simulink model "ProcessModel_Boeing1"  (Simulink 7.9)
settings: Solver=VariableStepDiscrete  StartTime=0.0  StopTime=inf  RelTol=1e-3
libraries: simeventslib x43, simulink x1
settings Model: Creator=tsprock3  LastModifiedBy=tsprock3
settings DebuggingCC: UnconnectedInputMsg=none  UnconnectedOutputMsg=none  SimStateOlderReleaseMsg=warning

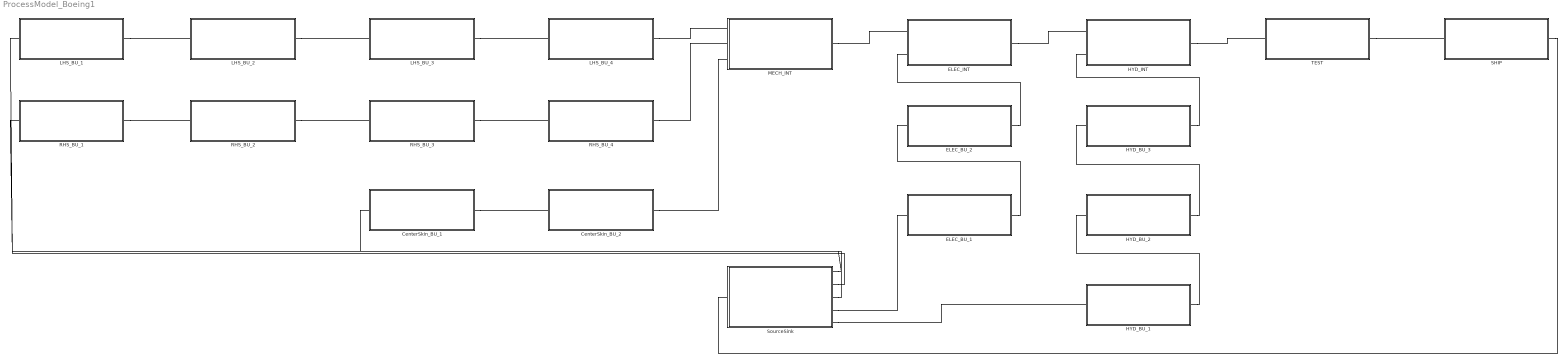
== system ProcessModel_Boeing1 ==
  CenterSkin_BU_1 : Subsystem
  CenterSkin_BU_2 : Subsystem
  ELEC_BU_1 : Subsystem
  ELEC_BU_2 : Subsystem
  ELEC_INT : Subsystem
  HYD_BU_1 : Subsystem
  HYD_BU_2 : Subsystem
  HYD_BU_3 : Subsystem
  HYD_INT : Subsystem
  LHS_BU_1 : Subsystem
  LHS_BU_2 : Subsystem
  LHS_BU_3 : Subsystem
  LHS_BU_4 : Subsystem
  MECH_INT : Subsystem
  RHS_BU_1 : Subsystem
  RHS_BU_2 : Subsystem
  RHS_BU_3 : Subsystem
  RHS_BU_4 : Subsystem
  SHIP : Subsystem
  SourceSink : Subsystem
  TEST : Subsystem
  connections:
  LHS_BU_1/RConn1 -- LHS_BU_2/LConn1
  LHS_BU_2/RConn1 -- LHS_BU_3/LConn1
  LHS_BU_3/RConn1 -- LHS_BU_4/LConn1
  RHS_BU_1/RConn1 -- RHS_BU_2/LConn1
  RHS_BU_2/RConn1 -- RHS_BU_3/LConn1
  RHS_BU_3/RConn1 -- RHS_BU_4/LConn1
  CenterSkin_BU_1/RConn1 -- CenterSkin_BU_2/LConn1
  LHS_BU_4/RConn1 -- MECH_INT/LConn1
  RHS_BU_4/RConn1 -- MECH_INT/LConn2
  CenterSkin_BU_2/RConn1 -- MECH_INT/LConn3
  MECH_INT/RConn1 -- ELEC_INT/LConn1
  ELEC_INT/RConn1 -- HYD_INT/LConn1
  ELEC_BU_1/RConn1 -- ELEC_BU_2/LConn1
  ELEC_BU_2/RConn1 -- ELEC_INT/LConn2
  HYD_BU_1/RConn1 -- HYD_BU_2/LConn1
  HYD_BU_2/RConn1 -- HYD_BU_3/LConn1
  HYD_BU_3/RConn1 -- HYD_INT/LConn2
  HYD_INT/RConn1 -- TEST/LConn1
  TEST/RConn1 -- SHIP/LConn1
  SourceSink/RConn1 -- LHS_BU_1/LConn1
  SourceSink/RConn2 -- RHS_BU_1/LConn1
  SourceSink/RConn3 -- CenterSkin_BU_1/LConn1
  SourceSink/RConn4 -- ELEC_BU_1/LConn1
  SourceSink/RConn5 -- HYD_BU_1/LConn1
  SHIP/RConn1 -- SourceSink/LConn1

== system ProcessModel_Boeing1/CenterSkin_BU_1 ==
  IN_Job : PathCombiner  NumberInputPorts=1
  OUT_Job : OutputSwitch  NumberOutputPorts=1
  Process : Subsystem
  IN_Job_1 : PMIOPort  Port=1  Side=Left
  OUT_Job_1 : PMIOPort  Port=2  Side=Right
  connections:
  Process/RConn1 -- OUT_Job/LConn1
  IN_Job/RConn1 -- Process/LConn1
  IN_Job/LConn1 -- IN_Job_1/RConn1
  OUT_Job/RConn1 -- OUT_Job_1/RConn1

== system ProcessModel_Boeing1/CenterSkin_BU_2 ==
  IN_Job : PathCombiner  NumberInputPorts=1
  OUT_Job : OutputSwitch  NumberOutputPorts=1
  Process : Subsystem
  IN_Job_1 : PMIOPort  Port=1  Side=Left
  OUT_Job_1 : PMIOPort  Port=2  Side=Right
  connections:
  Process/RConn1 -- OUT_Job/LConn1
  IN_Job/RConn1 -- Process/LConn1
  IN_Job/LConn1 -- IN_Job_1/RConn1
  OUT_Job/RConn1 -- OUT_Job_1/RConn1

== system ProcessModel_Boeing1/ELEC_BU_1 ==
  IN_Job : PathCombiner  NumberInputPorts=1
  OUT_Job : OutputSwitch  NumberOutputPorts=1
  Process : Subsystem
  IN_Job_1 : PMIOPort  Port=1  Side=Left
  OUT_Job_1 : PMIOPort  Port=2  Side=Right
  connections:
  Process/RConn1 -- OUT_Job/LConn1
  IN_Job/RConn1 -- Process/LConn1
  IN_Job/LConn1 -- IN_Job_1/RConn1
  OUT_Job/RConn1 -- OUT_Job_1/RConn1

== system ProcessModel_Boeing1/ELEC_BU_2 ==
  IN_Job : PathCombiner  NumberInputPorts=1
  OUT_Job : OutputSwitch  NumberOutputPorts=1
  Process : Subsystem
  IN_Job_1 : PMIOPort  Port=1  Side=Left
  OUT_Job_1 : PMIOPort  Port=2  Side=Right
  connections:
  Process/RConn1 -- OUT_Job/LConn1
  IN_Job/RConn1 -- Process/LConn1
  IN_Job/LConn1 -- IN_Job_1/RConn1
  OUT_Job/RConn1 -- OUT_Job_1/RConn1

== system ProcessModel_Boeing1/ELEC_INT ==
  IN_Job : EntityCombiner  NumberInputPorts=2  RetainComponentEntities=off
  OUT_Job : OutputSwitch  NumberOutputPorts=1
  Process : Subsystem
  IN_Job_1 : PMIOPort  Port=1  Side=Left
  IN_Job_2 : PMIOPort  Port=2  Side=Left
  OUT_Job_1 : PMIOPort  Port=3  Side=Right
  connections:
  Process/RConn1 -- OUT_Job/LConn1
  IN_Job/RConn1 -- Process/LConn1
  IN_Job/LConn1 -- IN_Job_1/RConn1
  IN_Job/LConn2 -- IN_Job_2/RConn1
  OUT_Job/RConn1 -- OUT_Job_1/RConn1

== system ProcessModel_Boeing1/HYD_BU_1 ==
  IN_Job : PathCombiner  NumberInputPorts=1
  OUT_Job : OutputSwitch  NumberOutputPorts=1
  Process : Subsystem
  IN_Job_1 : PMIOPort  Port=1  Side=Left
  OUT_Job_1 : PMIOPort  Port=2  Side=Right
  connections:
  Process/RConn1 -- OUT_Job/LConn1
  IN_Job/RConn1 -- Process/LConn1
  IN_Job/LConn1 -- IN_Job_1/RConn1
  OUT_Job/RConn1 -- OUT_Job_1/RConn1

== system ProcessModel_Boeing1/HYD_BU_2 ==
  IN_Job : PathCombiner  NumberInputPorts=1
  OUT_Job : OutputSwitch  NumberOutputPorts=1
  Process : Subsystem
  IN_Job_1 : PMIOPort  Port=1  Side=Left
  OUT_Job_1 : PMIOPort  Port=2  Side=Right
  connections:
  Process/RConn1 -- OUT_Job/LConn1
  IN_Job/RConn1 -- Process/LConn1
  IN_Job/LConn1 -- IN_Job_1/RConn1
  OUT_Job/RConn1 -- OUT_Job_1/RConn1

== system ProcessModel_Boeing1/HYD_BU_3 ==
  IN_Job : PathCombiner  NumberInputPorts=1
  OUT_Job : OutputSwitch  NumberOutputPorts=1
  Process : Subsystem
  IN_Job_1 : PMIOPort  Port=1  Side=Left
  OUT_Job_1 : PMIOPort  Port=2  Side=Right
  connections:
  Process/RConn1 -- OUT_Job/LConn1
  IN_Job/RConn1 -- Process/LConn1
  IN_Job/LConn1 -- IN_Job_1/RConn1
  OUT_Job/RConn1 -- OUT_Job_1/RConn1

== system ProcessModel_Boeing1/HYD_INT ==
  IN_Job : EntityCombiner  NumberInputPorts=2  RetainComponentEntities=off
  OUT_Job : OutputSwitch  NumberOutputPorts=1
  Process : Subsystem
  IN_Job_1 : PMIOPort  Port=1  Side=Left
  IN_Job_2 : PMIOPort  Port=2  Side=Left
  OUT_Job_1 : PMIOPort  Port=3  Side=Right
  connections:
  Process/RConn1 -- OUT_Job/LConn1
  IN_Job/RConn1 -- Process/LConn1
  IN_Job/LConn1 -- IN_Job_1/RConn1
  IN_Job/LConn2 -- IN_Job_2/RConn1
  OUT_Job/RConn1 -- OUT_Job_1/RConn1

== system ProcessModel_Boeing1/LHS_BU_1 ==
  IN_Job : PathCombiner  NumberInputPorts=1
  OUT_Job : OutputSwitch  NumberOutputPorts=1
  Process : Subsystem
  IN_Job_1 : PMIOPort  Port=1  Side=Left
  OUT_Job_1 : PMIOPort  Port=2  Side=Right
  connections:
  Process/RConn1 -- OUT_Job/LConn1
  IN_Job/RConn1 -- Process/LConn1
  IN_Job/LConn1 -- IN_Job_1/RConn1
  OUT_Job/RConn1 -- OUT_Job_1/RConn1

== system ProcessModel_Boeing1/LHS_BU_2 ==
  IN_Job : PathCombiner  NumberInputPorts=1
  OUT_Job : OutputSwitch  NumberOutputPorts=1
  Process : Subsystem
  IN_Job_1 : PMIOPort  Port=1  Side=Left
  OUT_Job_1 : PMIOPort  Port=2  Side=Right
  connections:
  Process/RConn1 -- OUT_Job/LConn1
  IN_Job/RConn1 -- Process/LConn1
  IN_Job/LConn1 -- IN_Job_1/RConn1
  OUT_Job/RConn1 -- OUT_Job_1/RConn1

== system ProcessModel_Boeing1/LHS_BU_3 ==
  IN_Job : PathCombiner  NumberInputPorts=1
  OUT_Job : OutputSwitch  NumberOutputPorts=1
  Process : Subsystem
  IN_Job_1 : PMIOPort  Port=1  Side=Left
  OUT_Job_1 : PMIOPort  Port=2  Side=Right
  connections:
  Process/RConn1 -- OUT_Job/LConn1
  IN_Job/RConn1 -- Process/LConn1
  IN_Job/LConn1 -- IN_Job_1/RConn1
  OUT_Job/RConn1 -- OUT_Job_1/RConn1

== system ProcessModel_Boeing1/LHS_BU_4 ==
  IN_Job : PathCombiner  NumberInputPorts=1
  OUT_Job : OutputSwitch  NumberOutputPorts=1
  Process : Subsystem
  IN_Job_1 : PMIOPort  Port=1  Side=Left
  OUT_Job_1 : PMIOPort  Port=2  Side=Right
  connections:
  Process/RConn1 -- OUT_Job/LConn1
  IN_Job/RConn1 -- Process/LConn1
  IN_Job/LConn1 -- IN_Job_1/RConn1
  OUT_Job/RConn1 -- OUT_Job_1/RConn1

== system ProcessModel_Boeing1/MECH_INT ==
  IN_Job : EntityCombiner  RetainComponentEntities=off
  OUT_Job : OutputSwitch  NumberOutputPorts=1
  Process : Subsystem
  IN_Job_1 : PMIOPort  Port=1  Side=Left
  IN_Job_2 : PMIOPort  Port=2  Side=Left
  IN_Job_3 : PMIOPort  Port=3  Side=Left
  OUT_Job_1 : PMIOPort  Port=4  Side=Right
  connections:
  Process/RConn1 -- OUT_Job/LConn1
  IN_Job/RConn1 -- Process/LConn1
  IN_Job/LConn1 -- IN_Job_1/RConn1
  IN_Job/LConn2 -- IN_Job_2/RConn1
  IN_Job/LConn3 -- IN_Job_3/RConn1
  OUT_Job/RConn1 -- OUT_Job_1/RConn1

== system ProcessModel_Boeing1/RHS_BU_1 ==
  IN_Job : PathCombiner  NumberInputPorts=1
  OUT_Job : OutputSwitch  NumberOutputPorts=1
  Process : Subsystem
  IN_Job_1 : PMIOPort  Port=1  Side=Left
  OUT_Job_1 : PMIOPort  Port=2  Side=Right
  connections:
  Process/RConn1 -- OUT_Job/LConn1
  IN_Job/RConn1 -- Process/LConn1
  IN_Job/LConn1 -- IN_Job_1/RConn1
  OUT_Job/RConn1 -- OUT_Job_1/RConn1

== system ProcessModel_Boeing1/RHS_BU_2 ==
  IN_Job : PathCombiner  NumberInputPorts=1
  OUT_Job : OutputSwitch  NumberOutputPorts=1
  Process : Subsystem
  IN_Job_1 : PMIOPort  Port=1  Side=Left
  OUT_Job_1 : PMIOPort  Port=2  Side=Right
  connections:
  Process/RConn1 -- OUT_Job/LConn1
  IN_Job/RConn1 -- Process/LConn1
  IN_Job/LConn1 -- IN_Job_1/RConn1
  OUT_Job/RConn1 -- OUT_Job_1/RConn1

== system ProcessModel_Boeing1/RHS_BU_3 ==
  IN_Job : PathCombiner  NumberInputPorts=1
  OUT_Job : OutputSwitch  NumberOutputPorts=1
  Process : Subsystem
  IN_Job_1 : PMIOPort  Port=1  Side=Left
  OUT_Job_1 : PMIOPort  Port=2  Side=Right
  connections:
  Process/RConn1 -- OUT_Job/LConn1
  IN_Job/RConn1 -- Process/LConn1
  IN_Job/LConn1 -- IN_Job_1/RConn1
  OUT_Job/RConn1 -- OUT_Job_1/RConn1

== system ProcessModel_Boeing1/RHS_BU_4 ==
  IN_Job : PathCombiner  NumberInputPorts=1
  OUT_Job : OutputSwitch  NumberOutputPorts=1
  Process : Subsystem
  IN_Job_1 : PMIOPort  Port=1  Side=Left
  OUT_Job_1 : PMIOPort  Port=2  Side=Right
  connections:
  Process/RConn1 -- OUT_Job/LConn1
  IN_Job/RConn1 -- Process/LConn1
  IN_Job/LConn1 -- IN_Job_1/RConn1
  OUT_Job/RConn1 -- OUT_Job_1/RConn1

== system ProcessModel_Boeing1/SHIP ==
  IN_Job : PathCombiner  NumberInputPorts=1
  OUT_Job : OutputSwitch  NumberOutputPorts=1
  Process : Subsystem
  IN_Job_1 : PMIOPort  Port=1  Side=Left
  OUT_Job_1 : PMIOPort  Port=2  Side=Right
  connections:
  Process/RConn1 -- OUT_Job/LConn1
  IN_Job/RConn1 -- Process/LConn1
  IN_Job/LConn1 -- IN_Job_1/RConn1
  OUT_Job/RConn1 -- OUT_Job_1/RConn1

== system ProcessModel_Boeing1/SourceSink ==
  IN_Job : EntityCombiner  NumberInputPorts=1  RetainComponentEntities=off
  OUT_Job : Replicate  NumberOutputPorts=5
  Process : Subsystem
  IN_Job_1 : PMIOPort  Port=1  Side=Left
  OUT_Job_1 : PMIOPort  Port=2  Side=Right
  OUT_Job_2 : PMIOPort  Port=3  Side=Right
  OUT_Job_3 : PMIOPort  Port=4  Side=Right
  OUT_Job_4 : PMIOPort  Port=5  Side=Right
  OUT_Job_5 : PMIOPort  Port=6  Side=Right
  connections:
  Process/RConn1 -- OUT_Job/LConn1
  IN_Job/RConn1 -- Process/LConn1
  IN_Job/LConn1 -- IN_Job_1/RConn1
  OUT_Job/RConn1 -- OUT_Job_1/RConn1
  OUT_Job/RConn2 -- OUT_Job_2/RConn1
  OUT_Job/RConn3 -- OUT_Job_3/RConn1
  OUT_Job/RConn4 -- OUT_Job_4/RConn1
  OUT_Job/RConn5 -- OUT_Job_5/RConn1

== system ProcessModel_Boeing1/TEST ==
  IN_Job : PathCombiner  NumberInputPorts=1
  OUT_Job : OutputSwitch  NumberOutputPorts=1
  Process : Subsystem
  IN_Job_1 : PMIOPort  Port=1  Side=Left
  OUT_Job_1 : PMIOPort  Port=2  Side=Right
  connections:
  Process/RConn1 -- OUT_Job/LConn1
  IN_Job/RConn1 -- Process/LConn1
  IN_Job/LConn1 -- IN_Job_1/RConn1
  OUT_Job/RConn1 -- OUT_Job_1/RConn1

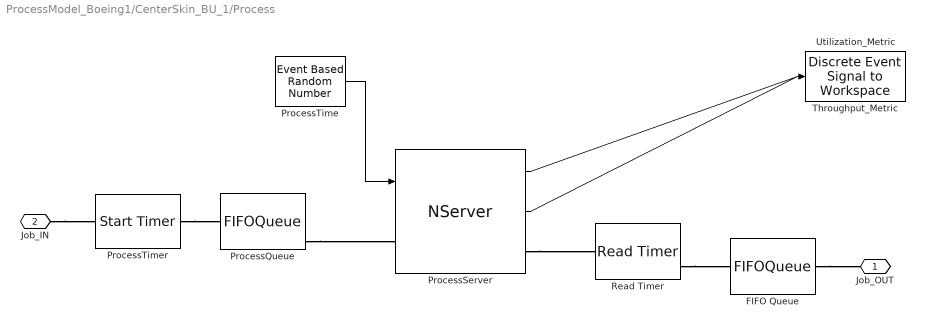
== system ProcessModel_Boeing1/CenterSkin_BU_1/Process ==
  FIFO Queue : FIFOQueue  Capacity=inf
  ProcessQueue : FIFOQueue  Capacity=inf  StatAverageWait=on  StatAverageQueueLength=on
      settings: OutputPortMap=o2,o3
  ProcessServer : NServer  NumberOfServers=6  ServiceTimeFrom=Signal port t  StatNumberDeparted=on  StatUtilization=on
      settings: OutputPortMap=o0,o5
  ProcessTime : EventBasedRandomNumber  Distribution=Gaussian (normal)  minUnif=1  meanNorm=4  stdNorm=0.4  Seed=19165
  ProcessTimer : StartTimer  TimerTag=T_CenterSkin_BU_1  TimerStartedOption=Restart
  Read Timer : ReadTimer  TimerTag=T_CenterSkin_BU_1  StatAverageTimeElapsed=on
      settings: OutputPortMap=o3
  Throughput_Metric : simeventslib/SimEvents Sinks/Discrete Event Signal to Workspace  VariableName=Throughput_CenterSkin_BU_1  SaveFormat=Structure With Time  isMonitorOnly=off  isRecordIC=off
  Utilization_Metric : simeventslib/SimEvents Sinks/Discrete Event Signal to Workspace  VariableName=Utilization_CenterSkin_BU_1  SaveFormat=Structure With Time  isMonitorOnly=off  isRecordIC=off
  Job_OUT : PMIOPort  Port=1  Side=Right
  Job_IN : PMIOPort  Port=2  Side=Left
  wires:
  ProcessTime/1 -> ProcessServer/1
  ProcessServer/1 -> Throughput_Metric/1
  ProcessServer/2 -> Utilization_Metric/1
  connections:
  FIFO Queue/RConn1 -- Job_OUT/RConn1
  Read Timer/RConn1 -- FIFO Queue/LConn1
  ProcessQueue/RConn1 -- ProcessServer/LConn1
  ProcessTimer/RConn1 -- ProcessQueue/LConn1
  ProcessServer/RConn1 -- Read Timer/LConn1
  Job_IN/RConn1 -- ProcessTimer/LConn1

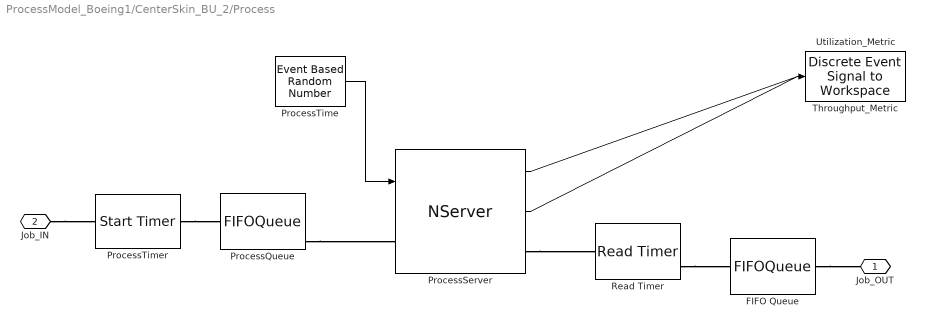
== system ProcessModel_Boeing1/CenterSkin_BU_2/Process ==
  FIFO Queue : FIFOQueue  Capacity=inf
  ProcessQueue : FIFOQueue  Capacity=inf  StatAverageWait=on  StatAverageQueueLength=on
      settings: OutputPortMap=o2,o3
  ProcessServer : NServer  NumberOfServers=9  ServiceTimeFrom=Signal port t  StatNumberDeparted=on  StatUtilization=on
      settings: OutputPortMap=o0,o5
  ProcessTime : EventBasedRandomNumber  Distribution=Gaussian (normal)  minUnif=1  meanNorm=5  stdNorm=0.5  Seed=22382
  ProcessTimer : StartTimer  TimerTag=T_CenterSkin_BU_2  TimerStartedOption=Restart
  Read Timer : ReadTimer  TimerTag=T_CenterSkin_BU_2  StatAverageTimeElapsed=on
      settings: OutputPortMap=o3
  Throughput_Metric : simeventslib/SimEvents Sinks/Discrete Event Signal to Workspace  VariableName=Throughput_CenterSkin_BU_2  SaveFormat=Structure With Time  isMonitorOnly=off  isRecordIC=off
  Utilization_Metric : simeventslib/SimEvents Sinks/Discrete Event Signal to Workspace  VariableName=Utilization_CenterSkin_BU_2  SaveFormat=Structure With Time  isMonitorOnly=off  isRecordIC=off
  Job_OUT : PMIOPort  Port=1  Side=Right
  Job_IN : PMIOPort  Port=2  Side=Left
  wires:
  ProcessTime/1 -> ProcessServer/1
  ProcessServer/1 -> Throughput_Metric/1
  ProcessServer/2 -> Utilization_Metric/1
  connections:
  FIFO Queue/RConn1 -- Job_OUT/RConn1
  Read Timer/RConn1 -- FIFO Queue/LConn1
  ProcessQueue/RConn1 -- ProcessServer/LConn1
  ProcessTimer/RConn1 -- ProcessQueue/LConn1
  ProcessServer/RConn1 -- Read Timer/LConn1
  Job_IN/RConn1 -- ProcessTimer/LConn1

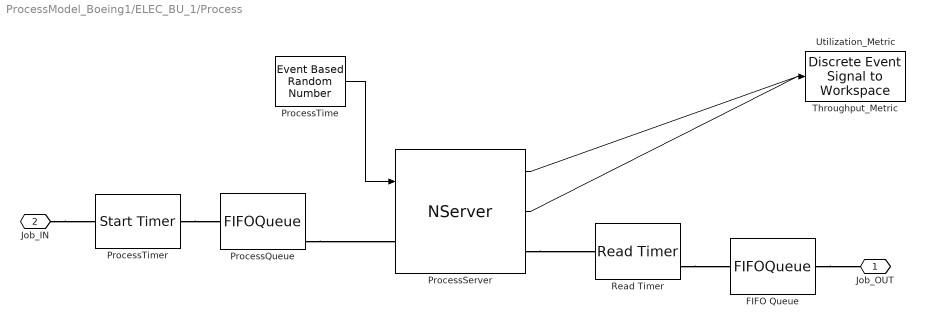
== system ProcessModel_Boeing1/ELEC_BU_1/Process ==
  FIFO Queue : FIFOQueue  Capacity=inf
  ProcessQueue : FIFOQueue  Capacity=inf  StatAverageWait=on  StatAverageQueueLength=on
      settings: OutputPortMap=o2,o3
  ProcessServer : NServer  ServiceTimeFrom=Signal port t  StatNumberDeparted=on  StatUtilization=on
      settings: OutputPortMap=o0,o5
  ProcessTime : EventBasedRandomNumber  Distribution=Gaussian (normal)  minUnif=1  meanNorm=4.5  stdNorm=0.45  Seed=25599
  ProcessTimer : StartTimer  TimerTag=T_ELEC_BU_1  TimerStartedOption=Restart
  Read Timer : ReadTimer  TimerTag=T_ELEC_BU_1  StatAverageTimeElapsed=on
      settings: OutputPortMap=o3
  Throughput_Metric : simeventslib/SimEvents Sinks/Discrete Event Signal to Workspace  VariableName=Throughput_ELEC_BU_1  SaveFormat=Structure With Time  isMonitorOnly=off  isRecordIC=off
  Utilization_Metric : simeventslib/SimEvents Sinks/Discrete Event Signal to Workspace  VariableName=Utilization_ELEC_BU_1  SaveFormat=Structure With Time  isMonitorOnly=off  isRecordIC=off
  Job_OUT : PMIOPort  Port=1  Side=Right
  Job_IN : PMIOPort  Port=2  Side=Left
  wires:
  ProcessTime/1 -> ProcessServer/1
  ProcessServer/1 -> Throughput_Metric/1
  ProcessServer/2 -> Utilization_Metric/1
  connections:
  FIFO Queue/RConn1 -- Job_OUT/RConn1
  Read Timer/RConn1 -- FIFO Queue/LConn1
  ProcessQueue/RConn1 -- ProcessServer/LConn1
  ProcessTimer/RConn1 -- ProcessQueue/LConn1
  ProcessServer/RConn1 -- Read Timer/LConn1
  Job_IN/RConn1 -- ProcessTimer/LConn1

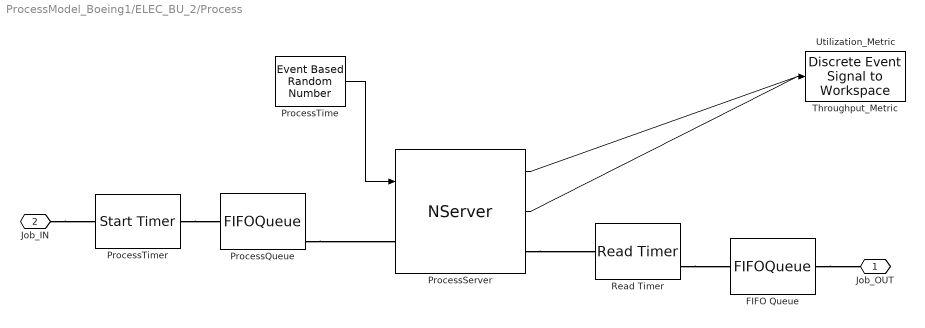
== system ProcessModel_Boeing1/ELEC_BU_2/Process ==
  FIFO Queue : FIFOQueue  Capacity=inf
  ProcessQueue : FIFOQueue  Capacity=inf  StatAverageWait=on  StatAverageQueueLength=on
      settings: OutputPortMap=o2,o3
  ProcessServer : NServer  ServiceTimeFrom=Signal port t  StatNumberDeparted=on  StatUtilization=on
      settings: OutputPortMap=o0,o5
  ProcessTime : EventBasedRandomNumber  Distribution=Gaussian (normal)  minUnif=1  meanNorm=4.5  stdNorm=0.45  Seed=28816
  ProcessTimer : StartTimer  TimerTag=T_ELEC_BU_2  TimerStartedOption=Restart
  Read Timer : ReadTimer  TimerTag=T_ELEC_BU_2  StatAverageTimeElapsed=on
      settings: OutputPortMap=o3
  Throughput_Metric : simeventslib/SimEvents Sinks/Discrete Event Signal to Workspace  VariableName=Throughput_ELEC_BU_2  SaveFormat=Structure With Time  isMonitorOnly=off  isRecordIC=off
  Utilization_Metric : simeventslib/SimEvents Sinks/Discrete Event Signal to Workspace  VariableName=Utilization_ELEC_BU_2  SaveFormat=Structure With Time  isMonitorOnly=off  isRecordIC=off
  Job_OUT : PMIOPort  Port=1  Side=Right
  Job_IN : PMIOPort  Port=2  Side=Left
  wires:
  ProcessTime/1 -> ProcessServer/1
  ProcessServer/1 -> Throughput_Metric/1
  ProcessServer/2 -> Utilization_Metric/1
  connections:
  FIFO Queue/RConn1 -- Job_OUT/RConn1
  Read Timer/RConn1 -- FIFO Queue/LConn1
  ProcessQueue/RConn1 -- ProcessServer/LConn1
  ProcessTimer/RConn1 -- ProcessQueue/LConn1
  ProcessServer/RConn1 -- Read Timer/LConn1
  Job_IN/RConn1 -- ProcessTimer/LConn1

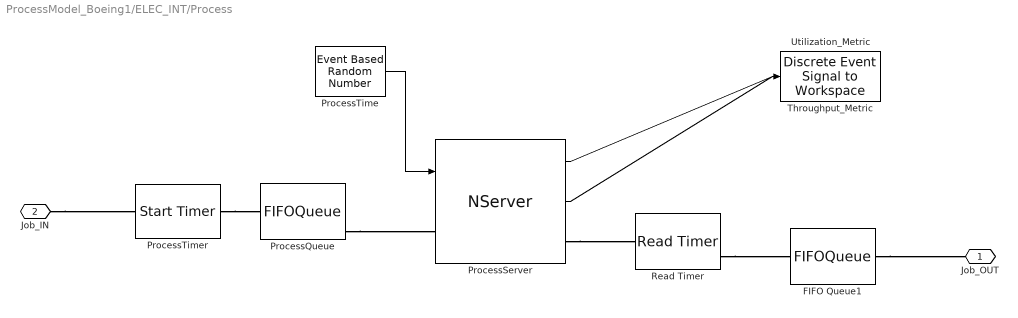
== system ProcessModel_Boeing1/ELEC_INT/Process ==
  FIFO Queue1 : FIFOQueue
  ProcessQueue : FIFOQueue  Capacity=inf  StatAverageWait=on  StatAverageQueueLength=on
      settings: OutputPortMap=o2,o3
  ProcessServer : NServer  NumberOfServers=7  ServiceTimeFrom=Signal port t  StatNumberDeparted=on  StatUtilization=on
      settings: OutputPortMap=o0,o5
  ProcessTime : EventBasedRandomNumber  Distribution=Gaussian (normal)  minUnif=1  meanNorm=6  stdNorm=0.6  Seed=32033
  ProcessTimer : StartTimer  TimerTag=T_ELEC_INT  TimerStartedOption=Restart
  Read Timer : ReadTimer  TimerTag=T_ELEC_INT  StatAverageTimeElapsed=on
      settings: OutputPortMap=o3
  Throughput_Metric : simeventslib/SimEvents Sinks/Discrete Event Signal to Workspace  VariableName=Throughput_ELEC_INT  SaveFormat=Structure With Time  isMonitorOnly=off  isRecordIC=off
  Utilization_Metric : simeventslib/SimEvents Sinks/Discrete Event Signal to Workspace  VariableName=Utilization_ELEC_INT  SaveFormat=Structure With Time  isMonitorOnly=off  isRecordIC=off
  Job_OUT : PMIOPort  Port=1  Side=Right
  Job_IN : PMIOPort  Port=2  Side=Left
  wires:
  ProcessTime/1 -> ProcessServer/1
  ProcessServer/1 -> Throughput_Metric/1
  ProcessServer/2 -> Utilization_Metric/1
  connections:
  FIFO Queue1/RConn1 -- Job_OUT/RConn1
  Read Timer/RConn1 -- FIFO Queue1/LConn1
  Job_IN/RConn1 -- ProcessTimer/LConn1
  ProcessQueue/RConn1 -- ProcessServer/LConn1
  ProcessTimer/RConn1 -- ProcessQueue/LConn1
  ProcessServer/RConn1 -- Read Timer/LConn1

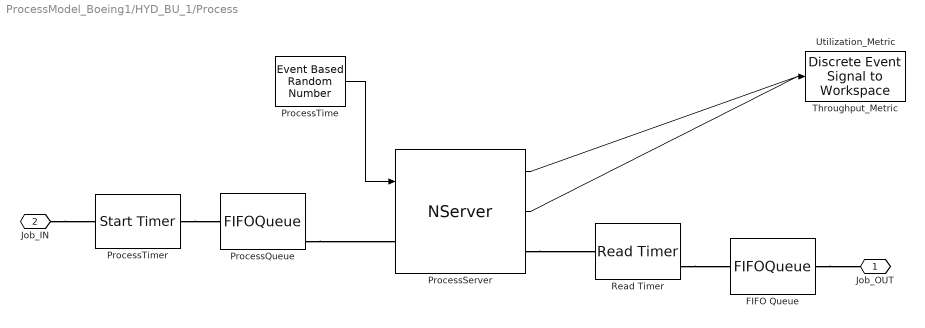
== system ProcessModel_Boeing1/HYD_BU_1/Process ==
  FIFO Queue : FIFOQueue  Capacity=inf
  ProcessQueue : FIFOQueue  Capacity=inf  StatAverageWait=on  StatAverageQueueLength=on
      settings: OutputPortMap=o2,o3
  ProcessServer : NServer  NumberOfServers=4  ServiceTimeFrom=Signal port t  StatNumberDeparted=on  StatUtilization=on
      settings: OutputPortMap=o0,o5
  ProcessTime : EventBasedRandomNumber  Distribution=Gaussian (normal)  minUnif=1  meanNorm=4  stdNorm=0.4  Seed=35250
  ProcessTimer : StartTimer  TimerTag=T_HYD_BU_1  TimerStartedOption=Restart
  Read Timer : ReadTimer  TimerTag=T_HYD_BU_1  StatAverageTimeElapsed=on
      settings: OutputPortMap=o3
  Throughput_Metric : simeventslib/SimEvents Sinks/Discrete Event Signal to Workspace  VariableName=Throughput_HYD_BU_1  SaveFormat=Structure With Time  isMonitorOnly=off  isRecordIC=off
  Utilization_Metric : simeventslib/SimEvents Sinks/Discrete Event Signal to Workspace  VariableName=Utilization_HYD_BU_1  SaveFormat=Structure With Time  isMonitorOnly=off  isRecordIC=off
  Job_OUT : PMIOPort  Port=1  Side=Right
  Job_IN : PMIOPort  Port=2  Side=Left
  wires:
  ProcessTime/1 -> ProcessServer/1
  ProcessServer/1 -> Throughput_Metric/1
  ProcessServer/2 -> Utilization_Metric/1
  connections:
  FIFO Queue/RConn1 -- Job_OUT/RConn1
  Read Timer/RConn1 -- FIFO Queue/LConn1
  ProcessQueue/RConn1 -- ProcessServer/LConn1
  ProcessTimer/RConn1 -- ProcessQueue/LConn1
  ProcessServer/RConn1 -- Read Timer/LConn1
  Job_IN/RConn1 -- ProcessTimer/LConn1

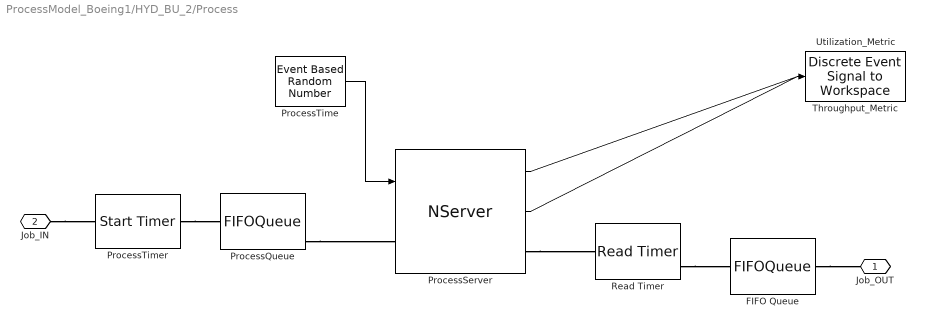
== system ProcessModel_Boeing1/HYD_BU_2/Process ==
  FIFO Queue : FIFOQueue  Capacity=inf
  ProcessQueue : FIFOQueue  Capacity=inf  StatAverageWait=on  StatAverageQueueLength=on
      settings: OutputPortMap=o2,o3
  ProcessServer : NServer  NumberOfServers=3  ServiceTimeFrom=Signal port t  StatNumberDeparted=on  StatUtilization=on
      settings: OutputPortMap=o0,o5
  ProcessTime : EventBasedRandomNumber  Distribution=Gaussian (normal)  minUnif=1  meanNorm=3  stdNorm=0.3  Seed=38467
  ProcessTimer : StartTimer  TimerTag=T_HYD_BU_2  TimerStartedOption=Restart
  Read Timer : ReadTimer  TimerTag=T_HYD_BU_2  StatAverageTimeElapsed=on
      settings: OutputPortMap=o3
  Throughput_Metric : simeventslib/SimEvents Sinks/Discrete Event Signal to Workspace  VariableName=Throughput_HYD_BU_2  SaveFormat=Structure With Time  isMonitorOnly=off  isRecordIC=off
  Utilization_Metric : simeventslib/SimEvents Sinks/Discrete Event Signal to Workspace  VariableName=Utilization_HYD_BU_2  SaveFormat=Structure With Time  isMonitorOnly=off  isRecordIC=off
  Job_OUT : PMIOPort  Port=1  Side=Right
  Job_IN : PMIOPort  Port=2  Side=Left
  wires:
  ProcessTime/1 -> ProcessServer/1
  ProcessServer/1 -> Throughput_Metric/1
  ProcessServer/2 -> Utilization_Metric/1
  connections:
  FIFO Queue/RConn1 -- Job_OUT/RConn1
  Read Timer/RConn1 -- FIFO Queue/LConn1
  ProcessQueue/RConn1 -- ProcessServer/LConn1
  ProcessTimer/RConn1 -- ProcessQueue/LConn1
  ProcessServer/RConn1 -- Read Timer/LConn1
  Job_IN/RConn1 -- ProcessTimer/LConn1

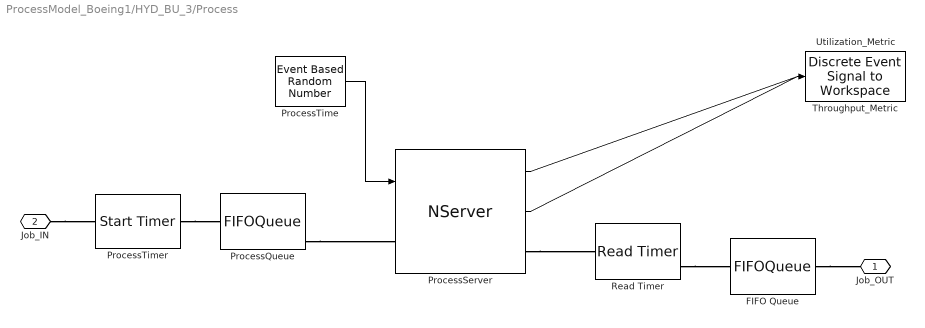
== system ProcessModel_Boeing1/HYD_BU_3/Process ==
  FIFO Queue : FIFOQueue  Capacity=inf
  ProcessQueue : FIFOQueue  Capacity=inf  StatAverageWait=on  StatAverageQueueLength=on
      settings: OutputPortMap=o2,o3
  ProcessServer : NServer  NumberOfServers=4  ServiceTimeFrom=Signal port t  StatNumberDeparted=on  StatUtilization=on
      settings: OutputPortMap=o0,o5
  ProcessTime : EventBasedRandomNumber  Distribution=Gaussian (normal)  minUnif=1  meanNorm=2  stdNorm=0.2  Seed=41684
  ProcessTimer : StartTimer  TimerTag=T_HYD_BU_3  TimerStartedOption=Restart
  Read Timer : ReadTimer  TimerTag=T_HYD_BU_3  StatAverageTimeElapsed=on
      settings: OutputPortMap=o3
  Throughput_Metric : simeventslib/SimEvents Sinks/Discrete Event Signal to Workspace  VariableName=Throughput_HYD_BU_3  SaveFormat=Structure With Time  isMonitorOnly=off  isRecordIC=off
  Utilization_Metric : simeventslib/SimEvents Sinks/Discrete Event Signal to Workspace  VariableName=Utilization_HYD_BU_3  SaveFormat=Structure With Time  isMonitorOnly=off  isRecordIC=off
  Job_OUT : PMIOPort  Port=1  Side=Right
  Job_IN : PMIOPort  Port=2  Side=Left
  wires:
  ProcessTime/1 -> ProcessServer/1
  ProcessServer/1 -> Throughput_Metric/1
  ProcessServer/2 -> Utilization_Metric/1
  connections:
  FIFO Queue/RConn1 -- Job_OUT/RConn1
  Read Timer/RConn1 -- FIFO Queue/LConn1
  ProcessQueue/RConn1 -- ProcessServer/LConn1
  ProcessTimer/RConn1 -- ProcessQueue/LConn1
  ProcessServer/RConn1 -- Read Timer/LConn1
  Job_IN/RConn1 -- ProcessTimer/LConn1

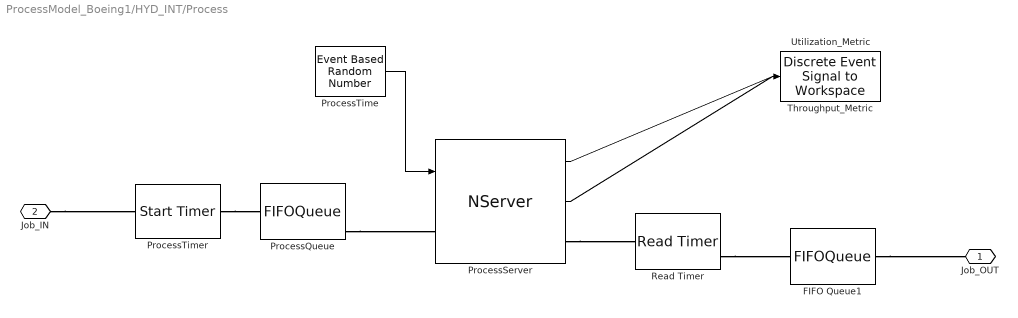
== system ProcessModel_Boeing1/HYD_INT/Process ==
  FIFO Queue1 : FIFOQueue
  ProcessQueue : FIFOQueue  Capacity=inf  StatAverageWait=on  StatAverageQueueLength=on
      settings: OutputPortMap=o2,o3
  ProcessServer : NServer  NumberOfServers=7  ServiceTimeFrom=Signal port t  StatNumberDeparted=on  StatUtilization=on
      settings: OutputPortMap=o0,o5
  ProcessTime : EventBasedRandomNumber  Distribution=Gaussian (normal)  minUnif=1  meanNorm=6  stdNorm=0.6  Seed=44901
  ProcessTimer : StartTimer  TimerTag=T_HYD_INT  TimerStartedOption=Restart
  Read Timer : ReadTimer  TimerTag=T_HYD_INT  StatAverageTimeElapsed=on
      settings: OutputPortMap=o3
  Throughput_Metric : simeventslib/SimEvents Sinks/Discrete Event Signal to Workspace  VariableName=Throughput_HYD_INT  SaveFormat=Structure With Time  isMonitorOnly=off  isRecordIC=off
  Utilization_Metric : simeventslib/SimEvents Sinks/Discrete Event Signal to Workspace  VariableName=Utilization_HYD_INT  SaveFormat=Structure With Time  isMonitorOnly=off  isRecordIC=off
  Job_OUT : PMIOPort  Port=1  Side=Right
  Job_IN : PMIOPort  Port=2  Side=Left
  wires:
  ProcessTime/1 -> ProcessServer/1
  ProcessServer/1 -> Throughput_Metric/1
  ProcessServer/2 -> Utilization_Metric/1
  connections:
  FIFO Queue1/RConn1 -- Job_OUT/RConn1
  Read Timer/RConn1 -- FIFO Queue1/LConn1
  Job_IN/RConn1 -- ProcessTimer/LConn1
  ProcessQueue/RConn1 -- ProcessServer/LConn1
  ProcessTimer/RConn1 -- ProcessQueue/LConn1
  ProcessServer/RConn1 -- Read Timer/LConn1

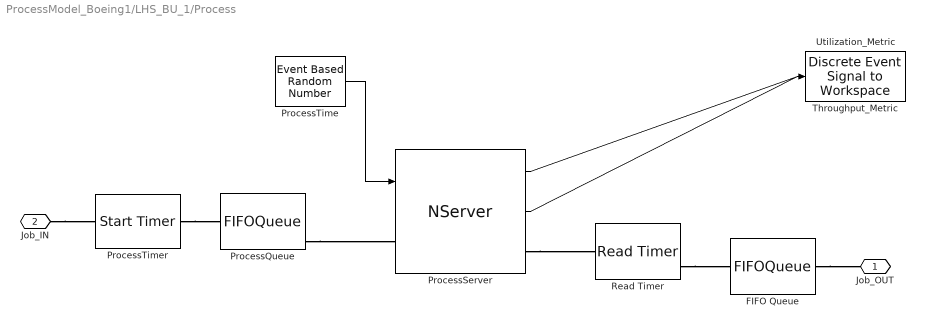
== system ProcessModel_Boeing1/LHS_BU_1/Process ==
  FIFO Queue : FIFOQueue  Capacity=inf
  ProcessQueue : FIFOQueue  Capacity=inf  StatAverageWait=on  StatAverageQueueLength=on
      settings: OutputPortMap=o2,o3
  ProcessServer : NServer  ServiceTimeFrom=Signal port t  StatNumberDeparted=on  StatUtilization=on
      settings: OutputPortMap=o0,o5
  ProcessTime : EventBasedRandomNumber  Distribution=Gaussian (normal)  minUnif=1  meanNorm=4  stdNorm=0.4  Seed=48118
  ProcessTimer : StartTimer  TimerTag=T_LHS_BU_1  TimerStartedOption=Restart
  Read Timer : ReadTimer  TimerTag=T_LHS_BU_1  StatAverageTimeElapsed=on
      settings: OutputPortMap=o3
  Throughput_Metric : simeventslib/SimEvents Sinks/Discrete Event Signal to Workspace  VariableName=Throughput_LHS_BU_1  SaveFormat=Structure With Time  isMonitorOnly=off  isRecordIC=off
  Utilization_Metric : simeventslib/SimEvents Sinks/Discrete Event Signal to Workspace  VariableName=Utilization_LHS_BU_1  SaveFormat=Structure With Time  isMonitorOnly=off  isRecordIC=off
  Job_OUT : PMIOPort  Port=1  Side=Right
  Job_IN : PMIOPort  Port=2  Side=Left
  wires:
  ProcessTime/1 -> ProcessServer/1
  ProcessServer/1 -> Throughput_Metric/1
  ProcessServer/2 -> Utilization_Metric/1
  connections:
  FIFO Queue/RConn1 -- Job_OUT/RConn1
  Read Timer/RConn1 -- FIFO Queue/LConn1
  ProcessQueue/RConn1 -- ProcessServer/LConn1
  ProcessTimer/RConn1 -- ProcessQueue/LConn1
  ProcessServer/RConn1 -- Read Timer/LConn1
  Job_IN/RConn1 -- ProcessTimer/LConn1

== system ProcessModel_Boeing1/LHS_BU_2/Process ==
  FIFO Queue : FIFOQueue  Capacity=inf
  ProcessQueue : FIFOQueue  Capacity=inf  StatAverageWait=on  StatAverageQueueLength=on
      settings: OutputPortMap=o2,o3
  ProcessServer : NServer  NumberOfServers=2  ServiceTimeFrom=Signal port t  StatNumberDeparted=on  StatUtilization=on
      settings: OutputPortMap=o0,o5
  ProcessTime : EventBasedRandomNumber  Distribution=Gaussian (normal)  minUnif=1  meanNorm=1  stdNorm=0.1  Seed=51335
  ProcessTimer : StartTimer  TimerTag=T_LHS_BU_2  TimerStartedOption=Restart
  Read Timer : ReadTimer  TimerTag=T_LHS_BU_2  StatAverageTimeElapsed=on
      settings: OutputPortMap=o3
  Throughput_Metric : simeventslib/SimEvents Sinks/Discrete Event Signal to Workspace  VariableName=Throughput_LHS_BU_2  SaveFormat=Structure With Time  isMonitorOnly=off  isRecordIC=off
  Utilization_Metric : simeventslib/SimEvents Sinks/Discrete Event Signal to Workspace  VariableName=Utilization_LHS_BU_2  SaveFormat=Structure With Time  isMonitorOnly=off  isRecordIC=off
  Job_OUT : PMIOPort  Port=1  Side=Right
  Job_IN : PMIOPort  Port=2  Side=Left
  wires:
  ProcessTime/1 -> ProcessServer/1
  ProcessServer/1 -> Throughput_Metric/1
  ProcessServer/2 -> Utilization_Metric/1
  connections:
  FIFO Queue/RConn1 -- Job_OUT/RConn1
  Read Timer/RConn1 -- FIFO Queue/LConn1
  ProcessQueue/RConn1 -- ProcessServer/LConn1
  ProcessTimer/RConn1 -- ProcessQueue/LConn1
  ProcessServer/RConn1 -- Read Timer/LConn1
  Job_IN/RConn1 -- ProcessTimer/LConn1

== system ProcessModel_Boeing1/LHS_BU_3/Process ==
  FIFO Queue : FIFOQueue  Capacity=inf
  ProcessQueue : FIFOQueue  Capacity=inf  StatAverageWait=on  StatAverageQueueLength=on
      settings: OutputPortMap=o2,o3
  ProcessServer : NServer  NumberOfServers=3  ServiceTimeFrom=Signal port t  StatNumberDeparted=on  StatUtilization=on
      settings: OutputPortMap=o0,o5
  ProcessTime : EventBasedRandomNumber  Distribution=Gaussian (normal)  minUnif=1  meanNorm=2  stdNorm=0.2  Seed=54552
  ProcessTimer : StartTimer  TimerTag=T_LHS_BU_3  TimerStartedOption=Restart
  Read Timer : ReadTimer  TimerTag=T_LHS_BU_3  StatAverageTimeElapsed=on
      settings: OutputPortMap=o3
  Throughput_Metric : simeventslib/SimEvents Sinks/Discrete Event Signal to Workspace  VariableName=Throughput_LHS_BU_3  SaveFormat=Structure With Time  isMonitorOnly=off  isRecordIC=off
  Utilization_Metric : simeventslib/SimEvents Sinks/Discrete Event Signal to Workspace  VariableName=Utilization_LHS_BU_3  SaveFormat=Structure With Time  isMonitorOnly=off  isRecordIC=off
  Job_OUT : PMIOPort  Port=1  Side=Right
  Job_IN : PMIOPort  Port=2  Side=Left
  wires:
  ProcessTime/1 -> ProcessServer/1
  ProcessServer/1 -> Throughput_Metric/1
  ProcessServer/2 -> Utilization_Metric/1
  connections:
  FIFO Queue/RConn1 -- Job_OUT/RConn1
  Read Timer/RConn1 -- FIFO Queue/LConn1
  ProcessQueue/RConn1 -- ProcessServer/LConn1
  ProcessTimer/RConn1 -- ProcessQueue/LConn1
  ProcessServer/RConn1 -- Read Timer/LConn1
  Job_IN/RConn1 -- ProcessTimer/LConn1

== system ProcessModel_Boeing1/LHS_BU_4/Process ==
  FIFO Queue : FIFOQueue  Capacity=inf
  ProcessQueue : FIFOQueue  Capacity=inf  StatAverageWait=on  StatAverageQueueLength=on
      settings: OutputPortMap=o2,o3
  ProcessServer : NServer  NumberOfServers=4  ServiceTimeFrom=Signal port t  StatNumberDeparted=on  StatUtilization=on
      settings: OutputPortMap=o0,o5
  ProcessTime : EventBasedRandomNumber  Distribution=Gaussian (normal)  minUnif=1  meanNorm=2  stdNorm=0.2  Seed=57769
  ProcessTimer : StartTimer  TimerTag=T_LHS_BU_4  TimerStartedOption=Restart
  Read Timer : ReadTimer  TimerTag=T_LHS_BU_4  StatAverageTimeElapsed=on
      settings: OutputPortMap=o3
  Throughput_Metric : simeventslib/SimEvents Sinks/Discrete Event Signal to Workspace  VariableName=Throughput_LHS_BU_4  SaveFormat=Structure With Time  isMonitorOnly=off  isRecordIC=off
  Utilization_Metric : simeventslib/SimEvents Sinks/Discrete Event Signal to Workspace  VariableName=Utilization_LHS_BU_4  SaveFormat=Structure With Time  isMonitorOnly=off  isRecordIC=off
  Job_OUT : PMIOPort  Port=1  Side=Right
  Job_IN : PMIOPort  Port=2  Side=Left
  wires:
  ProcessTime/1 -> ProcessServer/1
  ProcessServer/1 -> Throughput_Metric/1
  ProcessServer/2 -> Utilization_Metric/1
  connections:
  FIFO Queue/RConn1 -- Job_OUT/RConn1
  Read Timer/RConn1 -- FIFO Queue/LConn1
  ProcessQueue/RConn1 -- ProcessServer/LConn1
  ProcessTimer/RConn1 -- ProcessQueue/LConn1
  ProcessServer/RConn1 -- Read Timer/LConn1
  Job_IN/RConn1 -- ProcessTimer/LConn1

== system ProcessModel_Boeing1/MECH_INT/Process ==
  FIFO Queue1 : FIFOQueue
  ProcessQueue : FIFOQueue  Capacity=inf  StatAverageWait=on  StatAverageQueueLength=on
      settings: OutputPortMap=o2,o3
  ProcessServer : NServer  NumberOfServers=7  ServiceTimeFrom=Signal port t  StatNumberDeparted=on  StatUtilization=on
      settings: OutputPortMap=o0,o5
  ProcessTime : EventBasedRandomNumber  Distribution=Gaussian (normal)  minUnif=1  meanNorm=6  stdNorm=0.6  Seed=60986
  ProcessTimer : StartTimer  TimerTag=T_MECH_INT  TimerStartedOption=Restart
  Read Timer : ReadTimer  TimerTag=T_MECH_INT  StatAverageTimeElapsed=on
      settings: OutputPortMap=o3
  Throughput_Metric : simeventslib/SimEvents Sinks/Discrete Event Signal to Workspace  VariableName=Throughput_MECH_INT  SaveFormat=Structure With Time  isMonitorOnly=off  isRecordIC=off
  Utilization_Metric : simeventslib/SimEvents Sinks/Discrete Event Signal to Workspace  VariableName=Utilization_MECH_INT  SaveFormat=Structure With Time  isMonitorOnly=off  isRecordIC=off
  Job_OUT : PMIOPort  Port=1  Side=Right
  Job_IN : PMIOPort  Port=2  Side=Left
  wires:
  ProcessTime/1 -> ProcessServer/1
  ProcessServer/1 -> Throughput_Metric/1
  ProcessServer/2 -> Utilization_Metric/1
  connections:
  FIFO Queue1/RConn1 -- Job_OUT/RConn1
  Read Timer/RConn1 -- FIFO Queue1/LConn1
  Job_IN/RConn1 -- ProcessTimer/LConn1
  ProcessQueue/RConn1 -- ProcessServer/LConn1
  ProcessTimer/RConn1 -- ProcessQueue/LConn1
  ProcessServer/RConn1 -- Read Timer/LConn1

== system ProcessModel_Boeing1/RHS_BU_1/Process ==
  FIFO Queue : FIFOQueue  Capacity=inf
  ProcessQueue : FIFOQueue  Capacity=inf  StatAverageWait=on  StatAverageQueueLength=on
      settings: OutputPortMap=o2,o3
  ProcessServer : NServer  ServiceTimeFrom=Signal port t  StatNumberDeparted=on  StatUtilization=on
      settings: OutputPortMap=o0,o5
  ProcessTime : EventBasedRandomNumber  Distribution=Gaussian (normal)  minUnif=1  meanNorm=4  stdNorm=0.4  Seed=64203
  ProcessTimer : StartTimer  TimerTag=T_RHS_BU_1  TimerStartedOption=Restart
  Read Timer : ReadTimer  TimerTag=T_RHS_BU_1  StatAverageTimeElapsed=on
      settings: OutputPortMap=o3
  Throughput_Metric : simeventslib/SimEvents Sinks/Discrete Event Signal to Workspace  VariableName=Throughput_RHS_BU_1  SaveFormat=Structure With Time  isMonitorOnly=off  isRecordIC=off
  Utilization_Metric : simeventslib/SimEvents Sinks/Discrete Event Signal to Workspace  VariableName=Utilization_RHS_BU_1  SaveFormat=Structure With Time  isMonitorOnly=off  isRecordIC=off
  Job_OUT : PMIOPort  Port=1  Side=Right
  Job_IN : PMIOPort  Port=2  Side=Left
  wires:
  ProcessTime/1 -> ProcessServer/1
  ProcessServer/1 -> Throughput_Metric/1
  ProcessServer/2 -> Utilization_Metric/1
  connections:
  FIFO Queue/RConn1 -- Job_OUT/RConn1
  Read Timer/RConn1 -- FIFO Queue/LConn1
  ProcessQueue/RConn1 -- ProcessServer/LConn1
  ProcessTimer/RConn1 -- ProcessQueue/LConn1
  ProcessServer/RConn1 -- Read Timer/LConn1
  Job_IN/RConn1 -- ProcessTimer/LConn1

== system ProcessModel_Boeing1/RHS_BU_2/Process ==
  FIFO Queue : FIFOQueue  Capacity=inf
  ProcessQueue : FIFOQueue  Capacity=inf  StatAverageWait=on  StatAverageQueueLength=on
      settings: OutputPortMap=o2,o3
  ProcessServer : NServer  NumberOfServers=3  ServiceTimeFrom=Signal port t  StatNumberDeparted=on  StatUtilization=on
      settings: OutputPortMap=o0,o5
  ProcessTime : EventBasedRandomNumber  Distribution=Gaussian (normal)  minUnif=1  meanNorm=1  stdNorm=0.1  Seed=1884
  ProcessTimer : StartTimer  TimerTag=T_RHS_BU_2  TimerStartedOption=Restart
  Read Timer : ReadTimer  TimerTag=T_RHS_BU_2  StatAverageTimeElapsed=on
      settings: OutputPortMap=o3
  Throughput_Metric : simeventslib/SimEvents Sinks/Discrete Event Signal to Workspace  VariableName=Throughput_RHS_BU_2  SaveFormat=Structure With Time  isMonitorOnly=off  isRecordIC=off
  Utilization_Metric : simeventslib/SimEvents Sinks/Discrete Event Signal to Workspace  VariableName=Utilization_RHS_BU_2  SaveFormat=Structure With Time  isMonitorOnly=off  isRecordIC=off
  Job_OUT : PMIOPort  Port=1  Side=Right
  Job_IN : PMIOPort  Port=2  Side=Left
  wires:
  ProcessTime/1 -> ProcessServer/1
  ProcessServer/1 -> Throughput_Metric/1
  ProcessServer/2 -> Utilization_Metric/1
  connections:
  FIFO Queue/RConn1 -- Job_OUT/RConn1
  Read Timer/RConn1 -- FIFO Queue/LConn1
  ProcessQueue/RConn1 -- ProcessServer/LConn1
  ProcessTimer/RConn1 -- ProcessQueue/LConn1
  ProcessServer/RConn1 -- Read Timer/LConn1
  Job_IN/RConn1 -- ProcessTimer/LConn1

== system ProcessModel_Boeing1/RHS_BU_3/Process ==
  FIFO Queue : FIFOQueue  Capacity=inf
  ProcessQueue : FIFOQueue  Capacity=inf  StatAverageWait=on  StatAverageQueueLength=on
      settings: OutputPortMap=o2,o3
  ProcessServer : NServer  NumberOfServers=2  ServiceTimeFrom=Signal port t  StatNumberDeparted=on  StatUtilization=on
      settings: OutputPortMap=o0,o5
  ProcessTime : EventBasedRandomNumber  Distribution=Gaussian (normal)  minUnif=1  meanNorm=2  stdNorm=0.2  Seed=5101
  ProcessTimer : StartTimer  TimerTag=T_RHS_BU_3  TimerStartedOption=Restart
  Read Timer : ReadTimer  TimerTag=T_RHS_BU_3  StatAverageTimeElapsed=on
      settings: OutputPortMap=o3
  Throughput_Metric : simeventslib/SimEvents Sinks/Discrete Event Signal to Workspace  VariableName=Throughput_RHS_BU_3  SaveFormat=Structure With Time  isMonitorOnly=off  isRecordIC=off
  Utilization_Metric : simeventslib/SimEvents Sinks/Discrete Event Signal to Workspace  VariableName=Utilization_RHS_BU_3  SaveFormat=Structure With Time  isMonitorOnly=off  isRecordIC=off
  Job_OUT : PMIOPort  Port=1  Side=Right
  Job_IN : PMIOPort  Port=2  Side=Left
  wires:
  ProcessTime/1 -> ProcessServer/1
  ProcessServer/1 -> Throughput_Metric/1
  ProcessServer/2 -> Utilization_Metric/1
  connections:
  FIFO Queue/RConn1 -- Job_OUT/RConn1
  Read Timer/RConn1 -- FIFO Queue/LConn1
  ProcessQueue/RConn1 -- ProcessServer/LConn1
  ProcessTimer/RConn1 -- ProcessQueue/LConn1
  ProcessServer/RConn1 -- Read Timer/LConn1
  Job_IN/RConn1 -- ProcessTimer/LConn1

== system ProcessModel_Boeing1/RHS_BU_4/Process ==
  FIFO Queue : FIFOQueue  Capacity=inf
  ProcessQueue : FIFOQueue  Capacity=inf  StatAverageWait=on  StatAverageQueueLength=on
      settings: OutputPortMap=o2,o3
  ProcessServer : NServer  NumberOfServers=3  ServiceTimeFrom=Signal port t  StatNumberDeparted=on  StatUtilization=on
      settings: OutputPortMap=o0,o5
  ProcessTime : EventBasedRandomNumber  Distribution=Gaussian (normal)  minUnif=1  meanNorm=2  stdNorm=0.2  Seed=8318
  ProcessTimer : StartTimer  TimerTag=T_RHS_BU_4  TimerStartedOption=Restart
  Read Timer : ReadTimer  TimerTag=T_RHS_BU_4  StatAverageTimeElapsed=on
      settings: OutputPortMap=o3
  Throughput_Metric : simeventslib/SimEvents Sinks/Discrete Event Signal to Workspace  VariableName=Throughput_RHS_BU_4  SaveFormat=Structure With Time  isMonitorOnly=off  isRecordIC=off
  Utilization_Metric : simeventslib/SimEvents Sinks/Discrete Event Signal to Workspace  VariableName=Utilization_RHS_BU_4  SaveFormat=Structure With Time  isMonitorOnly=off  isRecordIC=off
  Job_OUT : PMIOPort  Port=1  Side=Right
  Job_IN : PMIOPort  Port=2  Side=Left
  wires:
  ProcessTime/1 -> ProcessServer/1
  ProcessServer/1 -> Throughput_Metric/1
  ProcessServer/2 -> Utilization_Metric/1
  connections:
  FIFO Queue/RConn1 -- Job_OUT/RConn1
  Read Timer/RConn1 -- FIFO Queue/LConn1
  ProcessQueue/RConn1 -- ProcessServer/LConn1
  ProcessTimer/RConn1 -- ProcessQueue/LConn1
  ProcessServer/RConn1 -- Read Timer/LConn1
  Job_IN/RConn1 -- ProcessTimer/LConn1

== system ProcessModel_Boeing1/SHIP/Process ==
  FIFO Queue : FIFOQueue  Capacity=inf
  ProcessQueue : FIFOQueue  Capacity=inf  StatAverageWait=on  StatAverageQueueLength=on
      settings: OutputPortMap=o2,o3
  ProcessServer : NServer  NumberOfServers=2  ServiceTimeFrom=Signal port t  StatNumberDeparted=on  StatUtilization=on
      settings: OutputPortMap=o0,o5
  ProcessTime : EventBasedRandomNumber  Distribution=Gaussian (normal)  minUnif=1  meanNorm=1  stdNorm=0.1  Seed=11535
  ProcessTimer : StartTimer  TimerTag=T_SHIP  TimerStartedOption=Restart
  Read Timer : ReadTimer  TimerTag=T_SHIP  StatAverageTimeElapsed=on
      settings: OutputPortMap=o3
  Throughput_Metric : simeventslib/SimEvents Sinks/Discrete Event Signal to Workspace  VariableName=Throughput_SHIP  SaveFormat=Structure With Time  isMonitorOnly=off  isRecordIC=off
  Utilization_Metric : simeventslib/SimEvents Sinks/Discrete Event Signal to Workspace  VariableName=Utilization_SHIP  SaveFormat=Structure With Time  isMonitorOnly=off  isRecordIC=off
  Job_OUT : PMIOPort  Port=1  Side=Right
  Job_IN : PMIOPort  Port=2  Side=Left
  wires:
  ProcessTime/1 -> ProcessServer/1
  ProcessServer/1 -> Throughput_Metric/1
  ProcessServer/2 -> Utilization_Metric/1
  connections:
  FIFO Queue/RConn1 -- Job_OUT/RConn1
  Read Timer/RConn1 -- FIFO Queue/LConn1
  ProcessQueue/RConn1 -- ProcessServer/LConn1
  ProcessTimer/RConn1 -- ProcessQueue/LConn1
  ProcessServer/RConn1 -- Read Timer/LConn1
  Job_IN/RConn1 -- ProcessTimer/LConn1

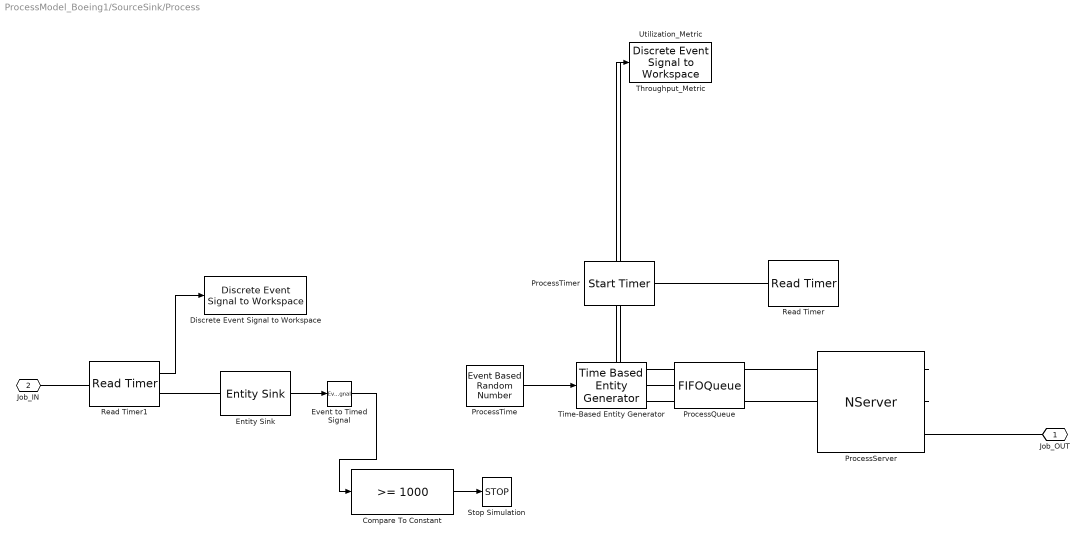
== system ProcessModel_Boeing1/SourceSink/Process ==
  Compare To Constant : simulink/Logic and Bit Operations/Compare To Constant  relop=>=  const=1000  OutDataTypeStr=boolean
  Discrete Event Signal to Workspace : simeventslib/SimEvents Sinks/Discrete Event Signal to Workspace  VariableName=ProcessTime  SaveFormat=Structure With Time  isMonitorOnly=off  isRecordIC=off
  Entity Sink : EntitySink  StatNumberArrived=on
  Event to Timed Signal : EventToTimedSignal
  ProcessQueue : FIFOQueue  Capacity=inf  StatAverageWait=on  StatAverageQueueLength=on
      settings: OutputPortMap=o2,o3
  ProcessServer : NServer  NumberOfServers=2  ServiceTime=0  StatNumberDeparted=on  StatUtilization=on
      settings: OutputPortMap=o0,o5
  ProcessTime : EventBasedRandomNumber  Distribution=Gaussian (normal)  minUnif=1  meanNorm=1  stdNorm=0.001  Seed=14752
  ProcessTimer : StartTimer  TimerTag=T_SourceSink  TimerStartedOption=Restart
  Read Timer : ReadTimer  TimerTag=T_SourceSink  StatAverageTimeElapsed=on
      settings: OutputPortMap=o3
  Read Timer1 : ReadTimer  TimerTag=T_LHS_BU_1  StatTimeElapsed=on
      settings: OutputPortMap=o2
  Stop Simulation : Stop
  Throughput_Metric : simeventslib/SimEvents Sinks/Discrete Event Signal to Workspace  VariableName=Throughput_SourceSink  SaveFormat=Structure With Time  isMonitorOnly=off  isRecordIC=off
  Time-Based Entity Generator : TimeBasedEntityGenerator  GenerateEntitiesUpon=Intergeneration time from port t
  Utilization_Metric : simeventslib/SimEvents Sinks/Discrete Event Signal to Workspace  VariableName=Utilization_SourceSink  SaveFormat=Structure With Time  isMonitorOnly=off  isRecordIC=off
  Job_OUT : PMIOPort  Port=1  Side=Right
  Job_IN : PMIOPort  Port=2  Side=Left
  wires:
  Entity Sink/1 -> Event to Timed Signal/1
  Event to Timed Signal/1 -> Compare To Constant/1
  Compare To Constant/1 -> Stop Simulation/1
  Read Timer1/1 -> Discrete Event Signal to Workspace/1
  ProcessTime/1 -> Time-Based Entity Generator/1
  ProcessServer/1 -> Throughput_Metric/1
  ProcessServer/2 -> Utilization_Metric/1
  connections:
  Job_IN/RConn1 -- Read Timer1/LConn1
  Read Timer1/RConn1 -- Entity Sink/LConn1
  ProcessServer/RConn1 -- Job_OUT/RConn1
  Time-Based Entity Generator/RConn1 -- ProcessQueue/LConn1
  ProcessTimer/RConn1 -- Read Timer/LConn1
  ProcessQueue/RConn1 -- ProcessServer/LConn1

== system ProcessModel_Boeing1/TEST/Process ==
  FIFO Queue : FIFOQueue  Capacity=inf
  ProcessQueue : FIFOQueue  Capacity=inf  StatAverageWait=on  StatAverageQueueLength=on
      settings: OutputPortMap=o2,o3
  ProcessServer : NServer  NumberOfServers=2  ServiceTimeFrom=Signal port t  StatNumberDeparted=on  StatUtilization=on
      settings: OutputPortMap=o0,o5
  ProcessTime : EventBasedRandomNumber  Distribution=Gaussian (normal)  minUnif=1  meanNorm=1  stdNorm=0.1  Seed=17969
  ProcessTimer : StartTimer  TimerTag=T_TEST  TimerStartedOption=Restart
  Read Timer : ReadTimer  TimerTag=T_TEST  StatAverageTimeElapsed=on
      settings: OutputPortMap=o3
  Throughput_Metric : simeventslib/SimEvents Sinks/Discrete Event Signal to Workspace  VariableName=Throughput_TEST  SaveFormat=Structure With Time  isMonitorOnly=off  isRecordIC=off
  Utilization_Metric : simeventslib/SimEvents Sinks/Discrete Event Signal to Workspace  VariableName=Utilization_TEST  SaveFormat=Structure With Time  isMonitorOnly=off  isRecordIC=off
  Job_OUT : PMIOPort  Port=1  Side=Right
  Job_IN : PMIOPort  Port=2  Side=Left
  wires:
  ProcessTime/1 -> ProcessServer/1
  ProcessServer/1 -> Throughput_Metric/1
  ProcessServer/2 -> Utilization_Metric/1
  connections:
  FIFO Queue/RConn1 -- Job_OUT/RConn1
  Read Timer/RConn1 -- FIFO Queue/LConn1
  ProcessQueue/RConn1 -- ProcessServer/LConn1
  ProcessTimer/RConn1 -- ProcessQueue/LConn1
  ProcessServer/RConn1 -- Read Timer/LConn1
  Job_IN/RConn1 -- ProcessTimer/LConn1
